simulink model "seldom_trim_sim"  (R2024a)
settings: Solver=VariableStepAuto  StartTime=0.0  StopTime=10.0  RelTol=1e-3  SampleTimeConstraint=STIndependent
undefined symbols (not defined in the file): Aircraft, Earth, Env, InitCond, WGS84
libraries: aerolibconvert2 x3, aerolibasang x3, simulink x2, aerolibatmos2 x1, vrlib x1, simulink_extras x1, spsLeadLagFilterLib x1, shared6dof x1, aerolibtransform2 x1, aerolibgravity2 x1
settings Model: Creator=brian  LastModifiedBy=joshb
settings SolverCC: AlgebraicLoopSolver=TrustRegion
settings DebuggingCC: UnconnectedInputMsg=warning  UnconnectedOutputMsg=warning  UnconnectedLineMsg=warning
settings ModelReferenceCC: EnableRefExpFcnMdlSchedulingChecks=on
settings RTWCC: GPUComputeCapability=3.5  DLArmComputeVersion=19.05

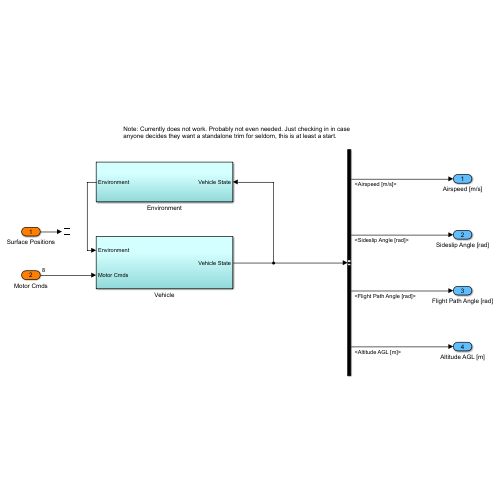
[thumbnail: Simulink's stored preview of the top-level diagram]
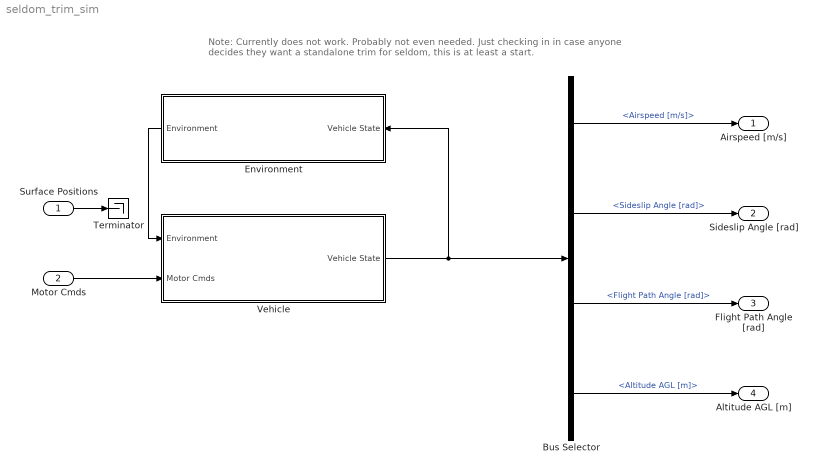
== system seldom_trim_sim ==
  note: Note: Currently does not work. Probably not even needed. Just checking in in case anyone decides they want a standalone trim for seldom, this is at least a start.
  Surface Positions : Inport
  Motor Cmds : Inport  Port=2  PortDimensions=Aircraft.Motor.nMotor
  Bus Selector : BusSelector  OutputSignals=Airspeed [m/s],Sideslip Angle [rad],Flight Path Angle [rad],Altitude AGL [m]
  Environment : Subsystem
  Terminator : Terminator
  Vehicle : Subsystem
  Airspeed [m/s] : Outport
  Sideslip Angle [rad] : Outport  Port=2
  Flight Path Angle [rad] : Outport  Port=3
  Altitude AGL [m] : Outport  Port=4
  wires:
  Vehicle/1(Vehicle State) -> Environment/1(Vehicle State), Bus Selector/1
  Environment/1(Environment) -> Vehicle/1(Environment)
  Surface Positions/1 -> Terminator/1
  Motor Cmds/1 -> Vehicle/2(Motor Cmds)
  Bus Selector/1 -> Airspeed [m/s]/1  "<Airspeed [m/s]>"
  Bus Selector/2 -> Sideslip Angle [rad]/1  "<Sideslip Angle [rad]>"
  Bus Selector/3 -> Flight Path Angle [rad]/1  "<Flight Path Angle [rad]>"
  Bus Selector/4 -> Altitude AGL [m]/1  "<Altitude AGL [m]>"

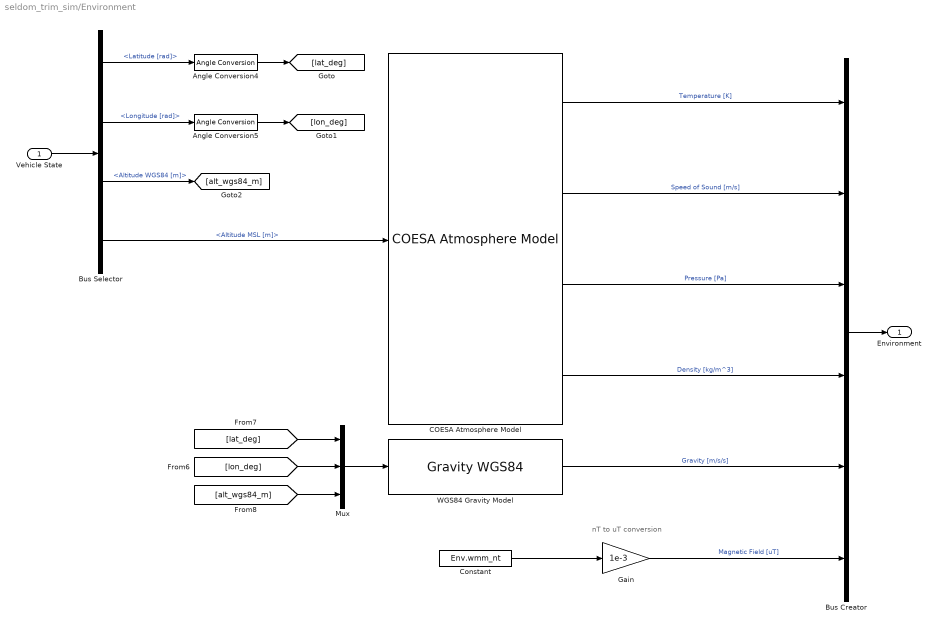
== system seldom_trim_sim/Environment ==
  note: nT to uT conversion
  Vehicle State : Inport
  Angle Conversion4 : aerolibconvert2/Angle Conversion  IU=rad  OU=deg
  Angle Conversion5 : aerolibconvert2/Angle Conversion  IU=rad  OU=deg
  Bus Creator : BusCreator  Inputs=6
  Bus Selector : BusSelector  OutputSignals=Latitude [rad],Longitude [rad],Altitude WGS84 [m],Altitude MSL [m]
  COESA Atmosphere Model : aerolibatmos2/COESA Atmosphere Model  units=Metric (MKS)  spec=1976 COESA-extended U.S. Standard Atmosphere  model=Profile  profile_var=High temperature  profile_percent=1%  profile_alt=5 km (16404 ft)  envelope_var=High temperature  envelope_percent=1%  action=Warning
  Constant : Constant  Value=Env.wmm_nt
  Gain : Gain  Gain=1e-3
  Mux : Mux  Inputs=3
  "WGS84 Gravity Model  " : GravityWGS84
  Environment : Outport
  wires:
  Angle Conversion5/1 -> [lon_deg]
  COESA Atmosphere Model/1 -> Bus Creator/1  "Temperature [K]"
  COESA Atmosphere Model/3 -> Bus Creator/3  "Pressure [Pa]"
  Bus Selector/1 -> Angle Conversion4/1  "<Latitude [rad]>"
  "WGS84 Gravity Model  "/1 -> Bus Creator/5  "Gravity [m/s/s]"
  Gain/1 -> Bus Creator/6  "Magnetic Field [uT]"
  Constant/1 -> Gain/1
  Bus Creator/1 -> Environment/1
  [lat_deg] -> Mux/1
  Angle Conversion4/1 -> [lat_deg]
  [alt_wgs84_m] -> Mux/3
  Bus Selector/4 -> COESA Atmosphere Model/1  "<Altitude MSL [m]>"
  COESA Atmosphere Model/2 -> Bus Creator/2  "Speed of Sound [m/s]"
  Bus Selector/2 -> Angle Conversion5/1  "<Longitude [rad]>"
  Vehicle State/1 -> Bus Selector/1
  Bus Selector/3 -> [alt_wgs84_m]  "<Altitude WGS84 [m]>"
  Mux/1 -> "WGS84 Gravity Model  "/1
  COESA Atmosphere Model/4 -> Bus Creator/4  "Density [kg/m^3]"
  [lon_deg] -> Mux/2

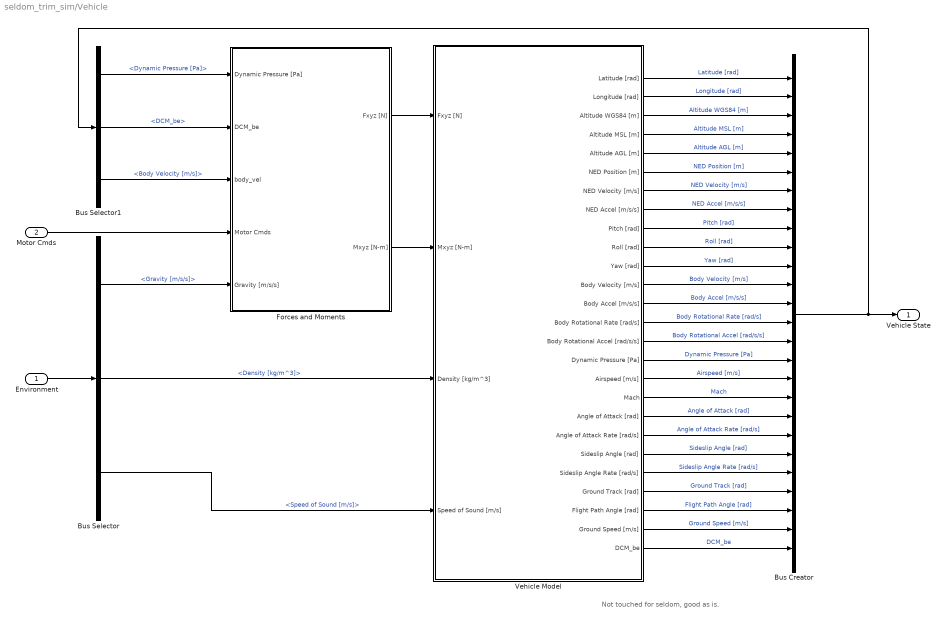
== system seldom_trim_sim/Vehicle ==
  note: Not touched for seldom, good as is.
  Environment : Inport
  Motor Cmds : Inport  Port=2
  Bus Creator : BusCreator  Inputs=26
  Bus Selector : BusSelector  OutputSignals=Gravity [m/s/s],Density [kg/m^3],Speed of Sound [m/s]
  Bus Selector1 : BusSelector  OutputSignals=Dynamic Pressure [Pa],DCM_be,Body Velocity [m/s]
  Forces and Moments : Subsystem
  Vehicle Model : Subsystem
  Vehicle State : Outport
  wires:
  Bus Selector1/3 -> Forces and Moments/3(body_vel)  "<Body Velocity [m/s]>"
  Vehicle Model/25(Ground Speed [m/s]) -> Bus Creator/25  "Ground Speed [m/s]"
  Vehicle Model/12(Body Velocity [m/s]) -> Bus Creator/12  "Body Velocity [m/s]"
  Vehicle Model/1(Latitude [rad]) -> Bus Creator/1  "Latitude [rad]"
  Vehicle Model/2(Longitude [rad]) -> Bus Creator/2  "Longitude [rad]"
  Motor Cmds/1 -> Forces and Moments/4(Motor Cmds)
  Vehicle Model/3(Altitude WGS84 [m]) -> Bus Creator/3  "Altitude WGS84 [m]"
  Vehicle Model/19(Angle of Attack [rad]) -> Bus Creator/19  "Angle of Attack [rad]"
  Forces and Moments/1(Fxyz [N]) -> Vehicle Model/1(Fxyz [N])
  Bus Creator/1 -> Vehicle State/1, Bus Selector1/1
  Bus Selector/3 -> Vehicle Model/4(Speed of Sound [m/s])  "<Speed of Sound [m/s]>"
  Environment/1 -> Bus Selector/1
  Forces and Moments/2(Mxyz [N-m]) -> Vehicle Model/2(Mxyz [N-m])
  Vehicle Model/8(NED Accel [m/s/s]) -> Bus Creator/8  "NED Accel [m/s/s]"
  Vehicle Model/9(Pitch [rad]) -> Bus Creator/9  "Pitch [rad]"
  Vehicle Model/13(Body Accel [m/s/s]) -> Bus Creator/13  "Body Accel [m/s/s]"
  Vehicle Model/14(Body Rotational Rate [rad/s]) -> Bus Creator/14  "Body Rotational Rate [rad/s]"
  Vehicle Model/15(Body Rotational Accel [rad/s/s]) -> Bus Creator/15  "Body Rotational Accel [rad/s/s]"
  Vehicle Model/17(Airspeed [m/s]) -> Bus Creator/17  "Airspeed [m/s]"
  Vehicle Model/7(NED Velocity [m/s]) -> Bus Creator/7  "NED Velocity [m/s]"
  Vehicle Model/10(Roll [rad]) -> Bus Creator/10  "Roll [rad]"
  Vehicle Model/23(Ground Track [rad]) -> Bus Creator/23  "Ground Track [rad]"
  Vehicle Model/6(NED Position [m]) -> Bus Creator/6  "NED Position [m]"
  Bus Selector/2 -> Vehicle Model/3(Density [kg/m^3])  "<Density [kg/m^3]>"
  Bus Selector1/2 -> Forces and Moments/2(DCM_be)  "<DCM_be>"
  Vehicle Model/5(Altitude AGL [m]) -> Bus Creator/5  "Altitude AGL [m]"
  Vehicle Model/18(Mach) -> Bus Creator/18  "Mach"
  Vehicle Model/11(Yaw [rad]) -> Bus Creator/11  "Yaw [rad]"
  Vehicle Model/24(Flight Path Angle [rad]) -> Bus Creator/24  "Flight Path Angle [rad]"
  Vehicle Model/21(Sideslip Angle [rad]) -> Bus Creator/21  "Sideslip Angle [rad]"
  Vehicle Model/22(Sideslip Angle Rate [rad/s]) -> Bus Creator/22  "Sideslip Angle Rate [rad/s]"
  Vehicle Model/16(Dynamic Pressure [Pa]) -> Bus Creator/16  "Dynamic Pressure [Pa]"
  Vehicle Model/26(DCM_be) -> Bus Creator/26  "DCM_be"
  Vehicle Model/4(Altitude MSL [m]) -> Bus Creator/4  "Altitude MSL [m]"
  Bus Selector1/1 -> Forces and Moments/1(Dynamic Pressure [Pa])  "<Dynamic Pressure [Pa]>"
  Vehicle Model/20(Angle of Attack Rate [rad/s]) -> Bus Creator/20  "Angle of Attack Rate [rad/s]"
  Bus Selector/1 -> Forces and Moments/5(Gravity [m/s/s])  "<Gravity [m/s/s]>"

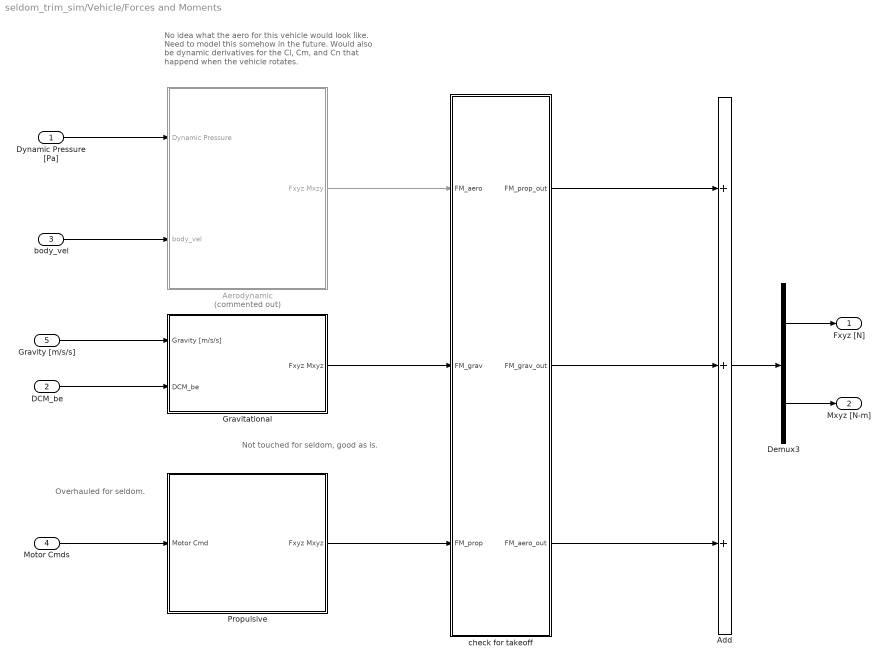
== system seldom_trim_sim/Vehicle/Forces and Moments ==
  note: Overhauled for seldom.
  note: No idea what the aero for this vehicle would look like. Need to model this somehow in the future. Would also be dynamic derivatives for the Cl, Cm, and Cn that happend when the vehicle rotates.
  note: Not touched for seldom, good as is.
  Dynamic Pressure [Pa] : Inport
  DCM_be : Inport  Port=2
  body_vel : Inport  Port=3
  Motor Cmds : Inport  Port=4
  Gravity [m/s/s] : Inport  Port=5
  Add : Sum  Inputs=+++
  Aerodynamic : Subsystem  Commented=on
  Demux3 : Demux  Outputs=2
  Gravitational : Subsystem
  Propulsive : Subsystem
  check for takeoff : Subsystem
  Fxyz [N] : Outport
  Mxyz [N-m] : Outport  Port=2
  wires:
  Propulsive/1(Fxyz Mxyz) -> check for takeoff/3(FM_prop)
  Aerodynamic/1(Fxyz Mxzy) -> check for takeoff/1(FM_aero)
  check for takeoff/3(FM_aero_out) -> Add/3
  check for takeoff/2(FM_grav_out) -> Add/2
  check for takeoff/1(FM_prop_out) -> Add/1
  Gravitational/1(Fxyz Mxyz) -> check for takeoff/2(FM_grav)
  body_vel/1 -> Aerodynamic/2(body_vel)
  Demux3/2 -> Mxyz [N-m]/1
  DCM_be/1 -> Gravitational/2(DCM_be)
  Dynamic Pressure [Pa]/1 -> Aerodynamic/1(Dynamic Pressure)
  Demux3/1 -> Fxyz [N]/1
  Motor Cmds/1 -> Propulsive/1(Motor Cmd)
  Gravity [m/s/s]/1 -> Gravitational/1(Gravity [m/s/s])
  Add/1 -> Demux3/1

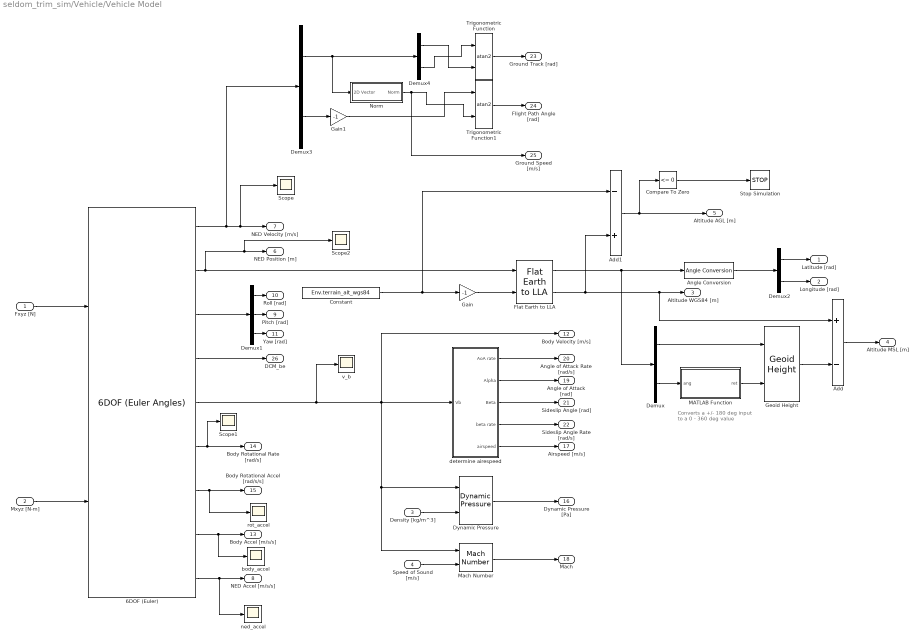
== system seldom_trim_sim/Vehicle/Vehicle Model ==
  note: Converts a +/- 180 deg
      | input to a 0 - 360 deg value
  Fxyz [N] : Inport
  Mxyz [N-m] : Inport  Port=2
  Density [kg/m^3] : Inport  Port=3
  Speed of Sound [m/s] : Inport  Port=4
  6DOF (Euler) : shared6dof/6DOF (Euler Angles)  units=Metric (MKS)  mtype=Fixed  rep=Euler Angles  xme_0=InitCond.ned_pos_m  Vm_0=InitCond.body_vel_mps  eul_0=InitCond.euler_rad  pm_0=InitCond.body_rot_rate_radps  mass_0=Aircraft.Mass.mass_kg  mass_e=0.5  mass_f=2.0  inertia=Aircraft.Mass.inertia_kgm2  inertia_e=eye(3)  inertia_f=2*eye(3)  k_quat=1.0  vre_flag=on  abi_flag=on  aMode=0  xme_statename=''  Vm_statename=''  eul_statename=''  quat_statename=''  pm_statename=''  mass_statename=''
  Add : Sum  Inputs=+-
  Add1 : Sum  Inputs=-+
  Angle Conversion : aerolibconvert2/Angle Conversion  IU=deg  OU=rad
  Compare To Zero : simulink/Logic and Bit Operations/Compare To Zero  relop=<=  OutDataTypeStr=boolean
  Constant : Constant  Value=Env.terrain_alt_wgs84
  Demux : Demux  Outputs=2
  Demux1 : Demux  Outputs=3
  Demux2 : Demux  Outputs=2
  Demux3 : Demux  Outputs=[2 1]
  Demux4 : Demux  Outputs=2
  Dynamic Pressure : aerolibasang/Dynamic Pressure
  Flat Earth to LLA : aerolibtransform2/Flat Earth to LLA  units=Metric (MKS)  ptype=Earth (WGS84)  F=1/298.257223563  R=6378137  refPosPort=off  LL0=[rad2deg(InitCond.lat_rad) rad2deg(InitCond.lon_rad)]  psi=0
  Gain : Gain  Gain=-1
  Gain1 : Gain  Gain=-1
  Geoid Height : aerolibgravity2/Geoid Height  units=Metric (MKS)  gtype=EGM2008  datafile='geoidegm96grid'  dtype=double  action=Warning
  MATLAB Function : MATLAB Function  TreatAsAtomicUnit=on
  Mach Number : aerolibasang/Mach Number
  Norm : Subsystem
  Scope : Scope
  Scope1 : Scope
  Scope2 : Scope
  Stop Simulation : Stop
  Trigonometric Function : Trigonometry  Operator=atan2
  Trigonometric Function1 : Trigonometry  Operator=atan2
  body_accel : Scope
  determine airespeed : Subsystem
  ned_accel : Scope
  rot_accel : Scope
  v_b : Scope
  Latitude [rad] : Outport
  Longitude [rad] : Outport  Port=2
  Altitude WGS84 [m] : Outport  Port=3
  Altitude MSL [m] : Outport  Port=4
  Altitude AGL [m] : Outport  Port=5
  NED Position [m] : Outport  Port=6
  NED Velocity [m/s] : Outport  Port=7
  NED Accel [m/s/s] : Outport  Port=8
  Pitch [rad] : Outport  Port=9
  Roll [rad] : Outport  Port=10
  Yaw [rad] : Outport  Port=11
  Body Velocity [m/s] : Outport  Port=12
  Body Accel [m/s/s] : Outport  Port=13
  Body Rotational Rate [rad/s] : Outport  Port=14
  Body Rotational Accel [rad/s/s] : Outport  Port=15
  Dynamic Pressure [Pa] : Outport  Port=16
  Airspeed [m/s] : Outport  Port=17
  Mach : Outport  Port=18
  Angle of Attack [rad] : Outport  Port=19
  Angle of Attack Rate [rad/s] : Outport  Port=20
  Sideslip Angle [rad] : Outport  Port=21
  Sideslip Angle Rate [rad/s] : Outport  Port=22
  Ground Track [rad] : Outport  Port=23
  Flight Path Angle [rad] : Outport  Port=24
  Ground Speed [m/s] : Outport  Port=25
  DCM_be : Outport  Port=26
  wires:
  Geoid Height/1 -> Add/2
  determine airespeed/5(airspeed) -> Airspeed [m/s]/1
  determine airespeed/4(beta rate) -> Sideslip Angle Rate [rad/s]/1
  determine airespeed/3(Beta) -> Sideslip Angle [rad]/1
  determine airespeed/2(Alpha) -> Angle of Attack [rad]/1
  determine airespeed/1(AoA rate) -> Angle of Attack Rate [rad/s]/1
  6DOF (Euler)/8 -> Body Accel [m/s/s]/1, body_accel/1
  Demux4/2 -> Trigonometric Function/1
  Demux4/1 -> Trigonometric Function/2
  Compare To Zero/1 -> Stop Simulation/1
  Add1/1 -> Altitude AGL [m]/1, Compare To Zero/1
  Constant/1 -> Gain/1, Add1/1
  Mach Number/1 -> Mach/1
  Speed of Sound [m/s]/1 -> Mach Number/2
  6DOF (Euler)/9 -> NED Accel [m/s/s]/1, ned_accel/1
  Trigonometric Function1/1 -> Flight Path Angle [rad]/1
  Norm/1(Norm) -> Trigonometric Function1/2, Ground Speed [m/s]/1
  Gain1/1 -> Trigonometric Function1/1
  Demux3/2 -> Gain1/1
  Trigonometric Function/1 -> Ground Track [rad]/1
  Demux3/1 -> Demux4/1, Norm/1(2D Vector)
  MATLAB Function/1(ret) -> Geoid Height/2
  6DOF (Euler)/1 -> NED Velocity [m/s]/1, Scope/1, Demux3/1
  6DOF (Euler)/7 -> Body Rotational Accel [rad/s/s]/1, rot_accel/1
  6DOF (Euler)/6 -> Body Rotational Rate [rad/s]/1, Scope1/1
  6DOF (Euler)/2 -> Flat Earth to LLA/1, NED Position [m]/1, Scope2/1
  Demux2/1 -> Latitude [rad]/1
  Demux2/2 -> Longitude [rad]/1
  Gain/1 -> Flat Earth to LLA/2
  Add/1 -> Altitude MSL [m]/1
  Dynamic Pressure/1 -> Dynamic Pressure [Pa]/1
  Demux1/3 -> Yaw [rad]/1
  Demux1/2 -> Pitch [rad]/1
  6DOF (Euler)/3 -> Demux1/1
  Demux1/1 -> Roll [rad]/1
  6DOF (Euler)/4 -> DCM_be/1
  Angle Conversion/1 -> Demux2/1
  Density [kg/m^3]/1 -> Dynamic Pressure/2
  Demux/1 -> Geoid Height/1
  Demux/2 -> MATLAB Function/1(ang)
  Flat Earth to LLA/2 -> Altitude WGS84 [m]/1, Add/1, Add1/2
  Flat Earth to LLA/1 -> Angle Conversion/1, Demux/1
  6DOF (Euler)/5 -> Body Velocity [m/s]/1, Mach Number/1, Dynamic Pressure/1, determine airespeed/1(Vb), v_b/1
  Mxyz [N-m]/1 -> 6DOF (Euler)/2
  Fxyz [N]/1 -> 6DOF (Euler)/1

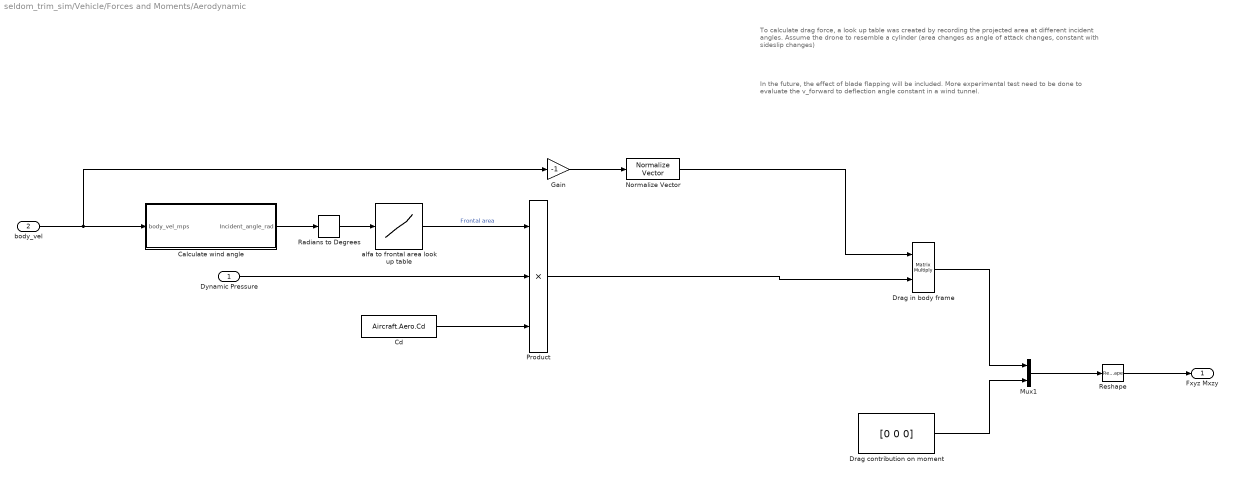
== system seldom_trim_sim/Vehicle/Forces and Moments/Aerodynamic ==
  note: To calculate drag force, a look up table was created by recording the projected area at different incident angles. Assume the drone to resemble a cylinder (area changes as angle of attack changes, constant with sideslip changes)
  note: In the future, the effect of blade flapping will be included. More experimental test need to be done to evaluate the v_forward to deflection angle constant in a wind tunnel.
  Dynamic Pressure : Inport
  body_vel : Inport  Port=2
  Calculate wind angle : Subsystem
  Cd : Constant  Value=Aircraft.Aero.Cd
  Drag contribution on moment : Constant  Value=[0 0 0]
  Drag in body frame : Product  Multiplication=Matrix(*)
  Gain : Gain  Gain=-1
  Mux1 : Mux  Inputs=2
  Normalize Vector : vrlib/Utilities/Normalize Vector  maxzero=0
  Product : Product  Inputs=3
  Radians to Degrees : simulink_extras/Transformations/Radians to Degrees
  Reshape : Reshape  OutputDimensionality=Row vector (2-D)
  alfa to frontal area look up table : Lookup_n-D  NumberOfTableDimensions=1  BreakpointsSpecification=Even spacing  BreakpointsForDimension1=[-90:10:90]  BreakpointsForDimension1FirstPoint=-180  BreakpointsForDimension1Spacing=10  Table=Aircraft.Geo.front_area_m2  InternalRulePriority=Speed  RndMeth=Simplest
  Fxyz Mxzy : Outport
  wires:
  Calculate wind angle/1(Incident_angle_rad) -> Radians to Degrees/1
  body_vel/1 -> Calculate wind angle/1(body_vel_mps), Gain/1
  Normalize Vector/1 -> Drag in body frame/1
  Gain/1 -> Normalize Vector/1
  Drag contribution on moment/1 -> Mux1/2
  Drag in body frame/1 -> Mux1/1
  Cd/1 -> Product/3
  alfa to frontal area look up table/1 -> Product/1  "Frontal area"
  Radians to Degrees/1 -> alfa to frontal area look up table/1
  Mux1/1 -> Reshape/1
  Reshape/1 -> Fxyz Mxzy/1
  Product/1 -> Drag in body frame/2
  Dynamic Pressure/1 -> Product/2

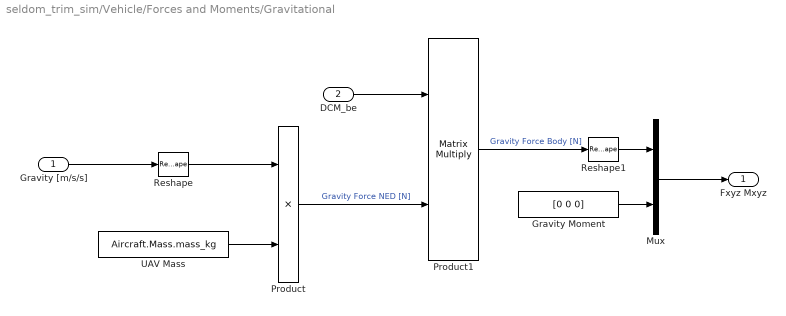
== system seldom_trim_sim/Vehicle/Forces and Moments/Gravitational ==
  Gravity [m/s/s] : Inport
  DCM_be : Inport  Port=2
  Gravity Moment : Constant  Value=[0 0 0]
  Mux : Mux  Inputs=2
  Product : Product
  Product1 : Product  Multiplication=Matrix(*)
  Reshape : Reshape  OutputDimensionality=Column vector (2-D)
  Reshape1 : Reshape
  UAV Mass : Constant  Value=Aircraft.Mass.mass_kg
  Fxyz Mxyz : Outport
  wires:
  Product1/1 -> Reshape1/1  "Gravity Force Body [N]"
  Reshape1/1 -> Mux/1
  Gravity [m/s/s]/1 -> Reshape/1
  Reshape/1 -> Product/1
  Mux/1 -> Fxyz Mxyz/1
  Gravity Moment/1 -> Mux/2
  DCM_be/1 -> Product1/1
  Product/1 -> Product1/2  "Gravity Force NED [N]"
  UAV Mass/1 -> Product/2

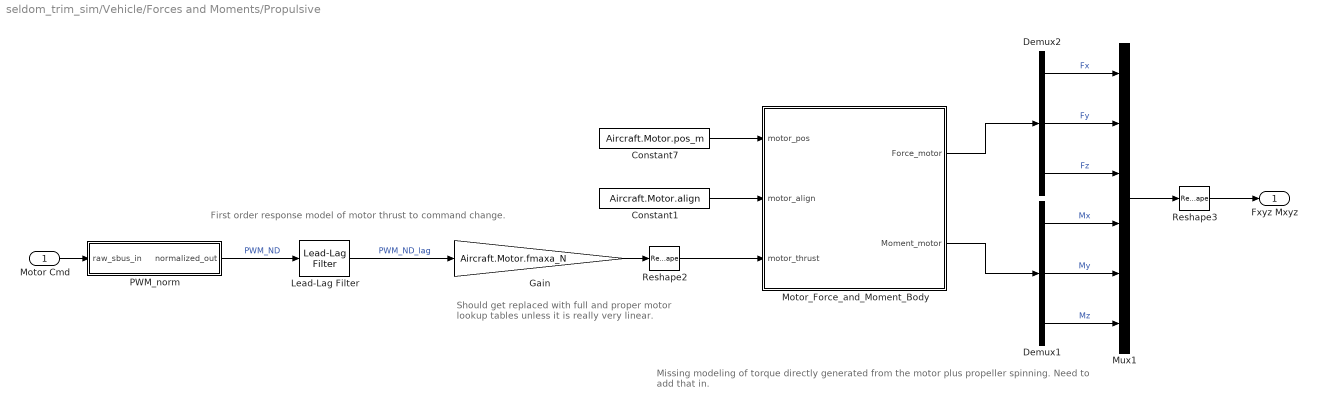
== system seldom_trim_sim/Vehicle/Forces and Moments/Propulsive ==
  note: First order response model of motor thrust to command change.
  note: Missing modeling of torque directly generated from the motor plus propeller spinning. Need to add that in.
  note: Should get replaced with full and proper motor lookup tables unless it is really very linear.
  Motor Cmd : Inport
  Constant1 : Constant  Value=Aircraft.Motor.align
  Constant7 : Constant  Value=Aircraft.Motor.pos_m
  Demux1 : Demux  Outputs=3
  Demux2 : Demux  Outputs=3
  Gain : Gain  Gain=Aircraft.Motor.fmaxa_N
  Lead-Lag Filter : spsLeadLagFilterLib/Lead-Lag Filter  T1=0  T2=Aircraft.Motor.Tau  Vdc_Init=0  Ts=0
      settings: LibrarySourceBlock=|
      | sps_lib/Control/Filters/Lead-Lag
      | Filter
  Motor_Force_and_Moment_Body : MATLAB Function  TreatAsAtomicUnit=on
  Mux1 : Mux  Inputs=6
  PWM_norm : Subsystem
  Reshape2 : Reshape  OutputDimensionality=Row vector (2-D)
  Reshape3 : Reshape  OutputDimensionality=Row vector (2-D)
  Fxyz Mxyz : Outport
  wires:
  PWM_norm/1(normalized_out) -> Lead-Lag Filter/1  "PWM_ND"
  Gain/1 -> Reshape2/1
  Lead-Lag Filter/1 -> Gain/1  "PWM_ND_lag"
  Motor_Force_and_Moment_Body/1(Force_motor) -> Demux2/1
  Demux2/3 -> Mux1/3  "Fz"
  Demux2/1 -> Mux1/1  "Fx"
  Demux2/2 -> Mux1/2  "Fy"
  Constant1/1 -> Motor_Force_and_Moment_Body/2(motor_align)
  Mux1/1 -> Reshape3/1
  Demux1/3 -> Mux1/6  "Mz"
  Reshape3/1 -> Fxyz Mxyz/1
  Constant7/1 -> Motor_Force_and_Moment_Body/1(motor_pos)
  Demux1/2 -> Mux1/5  "My"
  Demux1/1 -> Mux1/4  "Mx"
  Motor_Force_and_Moment_Body/2(Moment_motor) -> Demux1/1
  Motor Cmd/1 -> PWM_norm/1(raw_sbus_in)
  Reshape2/1 -> Motor_Force_and_Moment_Body/3(motor_thrust)

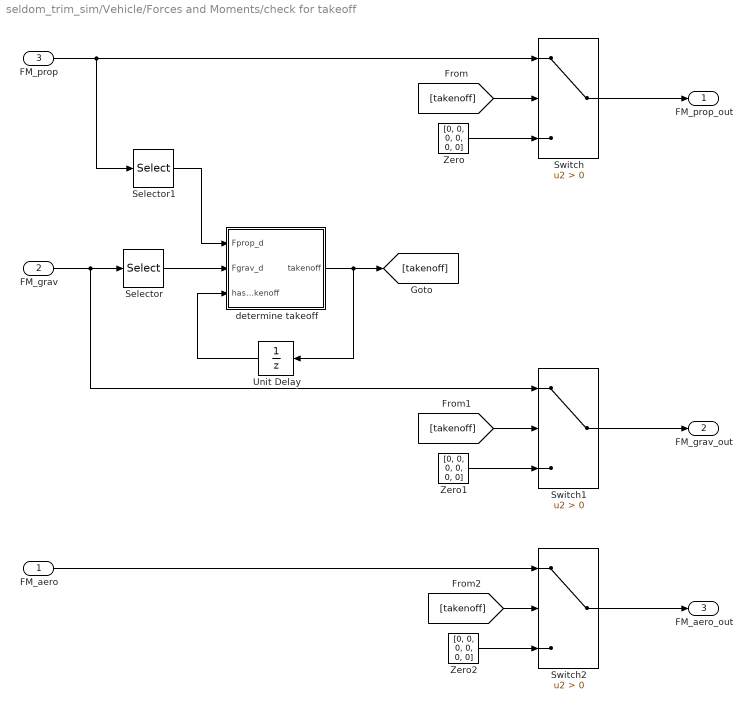
== system seldom_trim_sim/Vehicle/Forces and Moments/check for takeoff ==
  FM_aero : Inport
  FM_grav : Inport  Port=2
  FM_prop : Inport  Port=3
  Selector : Selector  NumberOfDimensions=2  InputPortWidth=3  IndexOptions=Index vector (dialog),Index vector (dialog)  Indices=1,3  OutputSizes=1,1
  Selector1 : Selector  NumberOfDimensions=2  InputPortWidth=3  IndexOptions=Index vector (dialog),Index vector (dialog)  Indices=1,3  OutputSizes=1,1
  Switch : Switch  Criteria=u2 > Threshold  SaturateOnIntegerOverflow=off  InputSameDT=off
  Switch1 : Switch  Criteria=u2 > Threshold  SaturateOnIntegerOverflow=off  InputSameDT=off
  Switch2 : Switch  Criteria=u2 > Threshold  SaturateOnIntegerOverflow=off  InputSameDT=off
  Unit Delay : UnitDelay  InitialCondition=false  SampleTime=-1  HasFrameUpgradeWarning=on
  Zero : Constant  Value=[0, 0, 0, 0, 0, 0]  VectorParams1D=off  OutDataTypeStr=Inherit: Inherit via back propagation
  Zero1 : Constant  Value=[0, 0, 0, 0, 0, 0]  VectorParams1D=off  OutDataTypeStr=Inherit: Inherit via back propagation
  Zero2 : Constant  Value=[0, 0, 0, 0, 0, 0]  VectorParams1D=off  OutDataTypeStr=Inherit: Inherit via back propagation
  determine takeoff : Subsystem
  FM_prop_out : Outport
  FM_grav_out : Outport  Port=2
  FM_aero_out : Outport  Port=3
  wires:
  Switch/1 -> FM_prop_out/1
  [takenoff] -> Switch2/2
  [takenoff] -> Switch/2
  Selector/1 -> determine takeoff/2(Fgrav_d)
  Zero/1 -> Switch/3
  Zero2/1 -> Switch2/3
  Zero1/1 -> Switch1/3
  determine takeoff/1(takenoff) -> Unit Delay/1, [takenoff]
  Unit Delay/1 -> determine takeoff/3(has_takenoff)
  FM_grav/1 -> Switch1/1, Selector/1
  Selector1/1 -> determine takeoff/1(Fprop_d)
  Switch1/1 -> FM_grav_out/1
  FM_aero/1 -> Switch2/1
  FM_prop/1 -> Switch/1, Selector1/1
  [takenoff] -> Switch1/2
  Switch2/1 -> FM_aero_out/1

== system seldom_trim_sim/Vehicle/Vehicle Model/Norm ==
  2D Vector : Inport
  Product : Product
  Sqrt : Sqrt
  Sum of Elements : Sum  Inputs=+
  Norm : Outport
  wires:
  Sqrt/1 -> Norm/1
  Sum of Elements/1 -> Sqrt/1
  Product/1 -> Sum of Elements/1
  2D Vector/1 -> Product/1, Product/2

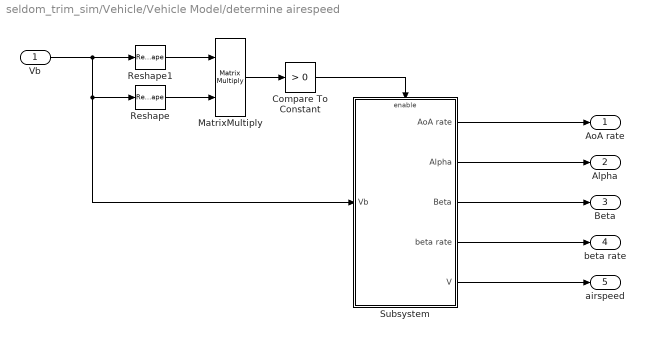
== system seldom_trim_sim/Vehicle/Vehicle Model/determine airespeed ==
  Vb : Inport
  Compare To Constant : simulink/Logic and Bit Operations/Compare To Constant  relop=>  const=0  OutDataTypeStr=boolean
  MatrixMultiply : Product  Multiplication=Matrix(*)
  Reshape : Reshape  OutputDimensionality=Column vector (2-D)
  Reshape1 : Reshape  OutputDimensionality=Row vector (2-D)
  Subsystem : Subsystem
  AoA rate : Outport
  Alpha : Outport  Port=2
  Beta : Outport  Port=3
  beta rate : Outport  Port=4
  airspeed : Outport  Port=5
  wires:
  Compare To Constant/1 -> Subsystem/Enable
  Subsystem/5(V) -> airspeed/1
  Subsystem/4(beta rate) -> beta rate/1
  Subsystem/3(Beta) -> Beta/1
  Subsystem/2(Alpha) -> Alpha/1
  Subsystem/1(AoA rate) -> AoA rate/1
  MatrixMultiply/1 -> Compare To Constant/1
  Reshape/1 -> MatrixMultiply/2
  Reshape1/1 -> MatrixMultiply/1
  Vb/1 -> Reshape1/1, Reshape/1, Subsystem/1(Vb)

== system seldom_trim_sim/Vehicle/Forces and Moments/Aerodynamic/Calculate wind angle ==
  body_vel_mps : Inport
  calculate_wind_angle : MATLAB Function  TreatAsAtomicUnit=on
  Incident_angle_rad : Outport
  wires:
  calculate_wind_angle/1(inc_ang) -> Incident_angle_rad/1
  body_vel_mps/1 -> calculate_wind_angle/1(body_vel)

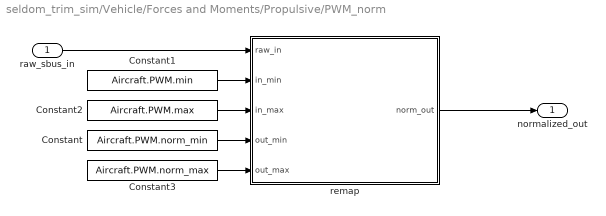
== system seldom_trim_sim/Vehicle/Forces and Moments/Propulsive/PWM_norm ==
  raw_sbus_in : Inport
  Constant : Constant  Value=Aircraft.PWM.norm_min  OutDataTypeStr=single
  Constant1 : Constant  Value=Aircraft.PWM.min  OutDataTypeStr=single
  Constant2 : Constant  Value=Aircraft.PWM.max  OutDataTypeStr=single
  Constant3 : Constant  Value=Aircraft.PWM.norm_max  OutDataTypeStr=single
  remap : MATLAB Function  TreatAsAtomicUnit=on
  normalized_out : Outport
  wires:
  raw_sbus_in/1 -> remap/1(raw_in)
  remap/1(norm_out) -> normalized_out/1
  Constant1/1 -> remap/2(in_min)
  Constant2/1 -> remap/3(in_max)
  Constant/1 -> remap/4(out_min)
  Constant3/1 -> remap/5(out_max)

== system seldom_trim_sim/Vehicle/Forces and Moments/check for takeoff/determine takeoff ==
  Fprop_d : Inport
  Fgrav_d : Inport  Port=2
  has_takenoff : Inport  Port=3
  Gain : Gain  Gain=-1
  GreaterThan : RelationalOperator  Operator=>  OutDataTypeStr=boolean  RndMeth=Simplest  InputSameDT=off
  OR : Logic  Operator=OR  IconShape=distinctive  AllPortsSameDT=off  OutDataTypeStr=boolean
  takenoff : Outport
  wires:
  OR/1 -> takenoff/1
  has_takenoff/1 -> OR/2
  GreaterThan/1 -> OR/1
  Gain/1 -> GreaterThan/1
  Fprop_d/1 -> Gain/1
  Fgrav_d/1 -> GreaterThan/2

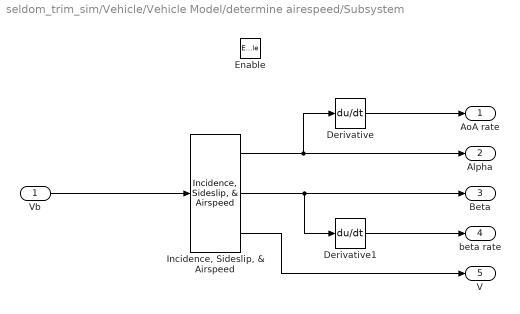
== system seldom_trim_sim/Vehicle/Vehicle Model/determine airespeed/Subsystem ==
  Vb : Inport
  Enable : EnablePort  StatesWhenEnabling=reset
  Derivative : Derivative
  Derivative1 : Derivative
  "Incidence, Sideslip, & Airspeed" : aerolibasang/Incidence, Sideslip, & Airspeed
  AoA rate : Outport
  Alpha : Outport  Port=2
  Beta : Outport  Port=3
  beta rate : Outport  Port=4
  V : Outport  Port=5
  wires:
  Derivative/1 -> AoA rate/1
  "Incidence, Sideslip, & Airspeed"/1 -> Derivative/1, Alpha/1
  "Incidence, Sideslip, & Airspeed"/3 -> V/1
  "Incidence, Sideslip, & Airspeed"/2 -> Derivative1/1, Beta/1
  Vb/1 -> "Incidence, Sideslip, & Airspeed"/1
  Derivative1/1 -> beta rate/1

== matlab function seldom_trim_sim/Vehicle/Vehicle Model/MATLAB Function ==
  data: ang input; ret output
function ret  = constrain360(ang)
%Constrain360 Converts a +/-180 value to a 0 - 360 value
ret = fmod(ang, 360);
if ret < 0
    ret = ret + 360;
end

end

== matlab function seldom_trim_sim/Vehicle/Forces and Moments/Aerodynamic/Calculate wind angle/calculate_wind_angle ==
  data: body_vel input; inc_ang output
function inc_ang = calculate_wind_angle(body_vel)

xy_mag = norm(body_vel(1:2));
if xy_mag > 0
    inc_ang = atan(xy_mag / body_vel(3));
else
    inc_ang = 0;
end

== matlab function seldom_trim_sim/Vehicle/Forces and Moments/Propulsive/Motor_Force_and_Moment_Body ==
  data: Force_motor output; motor_pos input; motor_align input; motor_thrust input; Moment_motor output
function [Force_motor,Moment_motor] = thrust_to_moment(motor_pos,motor_align,motor_thrust)
% Properly apply each motor's thrust to the correct orientation, then
% calculate the moment generated by each motor thrust
nmotor = numel(motor_thrust);
Force_motor_temp = zeros (nmotor,3);
Moment_motor_temp = zeros (nmotor,3);
for i = 1:nmotor
    Force_motor_temp(i,:) = motor_thrust(i)*motor_align(i,:); % F = T*normal_unit_vec
    Moment_motor_temp(i,:) = motor_thrust(i)*cross(motor_pos(i,:),motor_align(i,:)); % M = T*(pos-CG cross normal_unit_vec)
end
Force_motor  = sum (Force_motor_temp);
Moment_motor = sum (Moment_motor_temp);
end

== matlab function seldom_trim_sim/Vehicle/Forces and Moments/Propulsive/PWM_norm/remap ==
  data: raw_in input; norm_out output; in_min input; in_max input; out_min input; out_max input
function norm_out = remap(raw_in,in_min,in_max,out_min,out_max)
norm_out = (raw_in - in_min) * (out_max - out_min)/(in_max-in_min) + out_min;
